simulink model "connection4_first"  (R2017b)
settings: Solver=VariableStepAuto  StartTime=0.0  StopTime=50.0  RelTol=1e-3
values from neighbouring files (symbols this model uses):
  A4 = [-1,0,0,0,0,0,0,0,0,0 ... (first row only)    [param.m]
  D1_4 = [d1(1,1) ... (first row only)    [param.m]
  K1 = 1    [param.m]
  start = [0;1.5;0;-1.5;-3;3;-3;0;-3;-3]    [param.m]
settings Model: Creator=yunfei  LastModifiedBy=yunfei

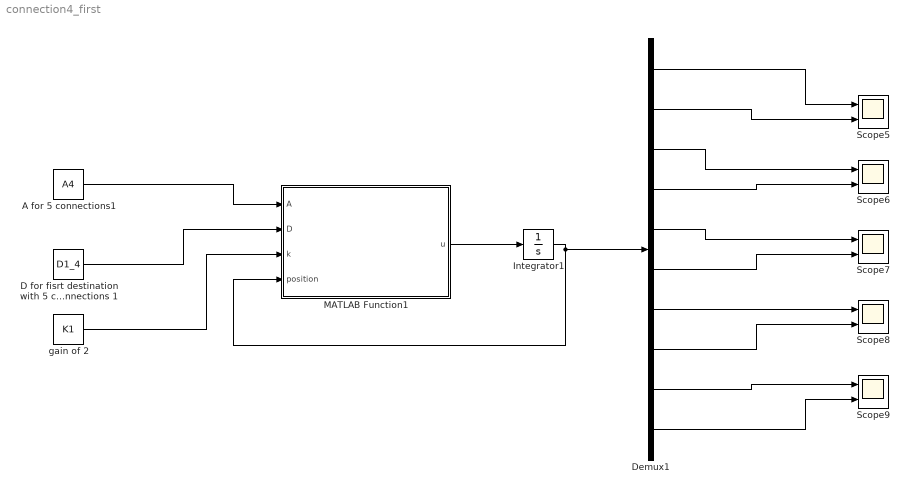
== system connection4_first ==
  A for 5 connections1 : Constant  Value=A4
  D for fisrt destination with 5 connections 1 : Constant  Value=D1_4
  Demux1 : Demux  Outputs=10
  Integrator1 : Integrator  InitialCondition=start
  MATLAB Function1 : MATLAB Function  TreatAsAtomicUnit=on
  Scope{5..9} (5 alike) : Scope  NumInputPorts=2
  gain of 2 : Constant  Value=K1
  wires:
  Demux1/6 -> Scope7/2
  Demux1/10 -> Scope9/2
  Demux1/8 -> Scope8/2
  Demux1/5 -> Scope7/1
  MATLAB Function1/1(u) -> Integrator1/1
  A for 5 connections1/1 -> MATLAB Function1/1(A)
  Demux1/4 -> Scope6/2
  Demux1/2 -> Scope5/2
  gain of 2/1 -> MATLAB Function1/3(k)
  Demux1/7 -> Scope8/1
  Demux1/3 -> Scope6/1
  Demux1/9 -> Scope9/1
  D for fisrt destination with 5 connections 1/1 -> MATLAB Function1/2(D)
  Demux1/1 -> Scope5/1
  Integrator1/1 -> MATLAB Function1/4(position), Demux1/1

== matlab function connection4_first/MATLAB Function1 ==
  data: A input; u output; D input; k input; position input
function u = fcn(A, D, k, position)
    u = k.*A * position + D;
end
